simulink model "model"  (R2014a)
settings: Solver=FixedStepDiscrete  StartTime=0.0  StopTime=10  RelTol=1e-3
values from neighbouring files (symbols this model uses):
  BufLen = 4*Fs    [init_model.m]
  delay_fp1 = ceil(delay_qrs-fpdl-fpdi-fpdd)    [init_model.m]
  delay_fp2 = ceil(delay_qrs-fpdl-s)    [init_model.m]
  delay_noise = ceil(noiseds + noisedl)    [init_model.m]
  Fs = signal.fs    [init_model.m]
  s = round(0.06*Fs)    [init_model.m]
undefined symbols (not defined in the file or in its folder): fpad, fpai, fpal, fpbd, fpbi, fpbl, FrameLen, get, gopalakhermite, HR, JayMeasurePts, noiseal, noiseas, noisebl, noisebs, qrsad, qrsah, qrsai, qrsal, qrsbd, qrsbh, qrsbi, qrsbl, qrsgh, qrsgl, rochahermite1, rochahermite2, stlen
undefined symbols (not defined in the file): L1, L2, L3, L4, newL1, newL2
libraries: simulink x16, neural x14, dspbuff3 x4, dspsigops x2, dspsnks4 x1
(part 2 of 2)

== system model/Classification/Rocha Networks/Feed-Forward Neural Network/Layer 1/Delays 1 ==
  "p{1}" : Inport  PortDimensions=14  SampleTime=0.004
      mask Display: e = 0.06;c1 = [120 230 180]/255;c2 = ([120 230 180]+0)/(256+128);c3 = ([120 230 180]+128)/(256+128);patch([0 1 1 0],[0 0 1 1],c1);patch([0 1 1 1-e 1-e 0+e],[0 0 1 1-e 0+e 0+e],c2);patch([0 0 1 1-e 0+e 0+e],[0 1 1 1-e 1-e 0+e],c3);plot([0 1 1 0 0],[0 0 1 1 0]);
  mux : Mux  Inputs=1
      mask Display: e = 0.06;c1 = [120 150 230]/255;c2 = ([120 150 230]+0)/383;c3 = ([120 150 230]+128)/383;patch([0 1 1 0],[0 0 1 1],c1);patch([0 1 1 1-e 1-e 0+e],[0 0 1 1-e 0+e 0+e],c2);patch([0 0 1 1-e 0+e 0+e],[0 1 1 1-e 1-e 0+e],c3);plot([0 1 1 0 0],[0 0 1 1 0]);disp('Mux')
  "pd{1,1}" : Outport
      mask Display: e = 0.06;c1 = [120 230 180]/255;c2 = ([120 230 180]+0)/(256+128);c3 = ([120 230 180]+128)/(256+128);patch([0 1 1 0],[0 0 1 1],c1);patch([0 1 1 1-e 1-e 0+e],[0 0 1 1-e 0+e 0+e],c2);patch([0 0 1 1-e 0+e 0+e],[0 1 1 1-e 1-e 0+e],c3);plot([0 1 1 0 0],[0 0 1 1 0]);
  wires:
  mux/1 -> "pd{1,1}"/1
  "p{1}"/1 -> mux/1

== system model/Classification/Rocha Networks/Feed-Forward Neural Network/Layer 1/IW{1,1} ==
  "pd{1,1}" : Inport  PortDimensions=14  SampleTime=0.004
      mask Display: e = 0.06;c1 = [120 230 180]/255;c2 = ([120 230 180]+0)/(256+128);c3 = ([120 230 180]+128)/(256+128);patch([0 1 1 0],[0 0 1 1],c1);patch([0 1 1 1-e 1-e 0+e],[0 0 1 1-e 0+e 0+e],c2);patch([0 0 1 1-e 0+e 0+e],[0 1 1 1-e 1-e 0+e],c3);plot([0 1 1 0 0],[0 0 1 1 0]);
  "IW{1,1}(1,:)'" : Constant  Value=[-0.94852743044432697;0.20440062307916493;0.12975491445977652;-0.06056239618675234;0.069962133679617386;-0.10885123721830199;0.25849498473889437;-0.053514204484363927;-0.25705609193888052;-0.26702768869811228;-0.044345977422213696;-0.355114180368993;0.3456890098950946;0.33374461628287727]
      mask Display: e = 0.06;c1 = [120 150 230]/255;c2 = ([120 150 230]+0)/383;c3 = ([120 150 230]+128)/383;patch([0 1 1 0],[0 0 1 1],c1);patch([0 1 1 1-e 1-e 0+e],[0 0 1 1-e 0+e 0+e],c2);patch([0 0 1 1-e 0+e 0+e],[0 1 1 1-e 1-e 0+e],c3);plot([0 1 1 0 0],[0 0 1 1 0]);disp('Weights');
  "IW{1,1}(2,:)'" : Constant  Value=[4.196215953221297;-1.0964533347848004;-1.6910456916650782;1.1678044277703084;-0.91890034705408374;-1.3729579966623704;-1.6439744697625485;-1.20511805638854;-7.3755359553788633;2.9486890292671837;2.0933673220936755;-1.7229669045940939;5.0896314895005839;2.1588793540686324]
      mask Display: e = 0.06;c1 = [120 150 230]/255;c2 = ([120 150 230]+0)/383;c3 = ([120 150 230]+128)/383;patch([0 1 1 0],[0 0 1 1],c1);patch([0 1 1 1-e 1-e 0+e],[0 0 1 1-e 0+e 0+e],c2);patch([0 0 1 1-e 0+e 0+e],[0 1 1 1-e 1-e 0+e],c3);plot([0 1 1 0 0],[0 0 1 1 0]);disp('Weights');
  "IW{1,1}(3,:)'" : Constant  Value=[-119.48893768603425;100.34105004135291;-30.003324500089562;-35.099277290990273;-53.005837073603445;50.742281662417867;-89.637475943048045;20.647748261081514;-41.338537083861603;-272.57547073663108;116.09637700457249;-23.032516013581716;83.319718635034363;79.324095644747445]
      mask Display: e = 0.06;c1 = [120 150 230]/255;c2 = ([120 150 230]+0)/383;c3 = ([120 150 230]+128)/383;patch([0 1 1 0],[0 0 1 1],c1);patch([0 1 1 1-e 1-e 0+e],[0 0 1 1-e 0+e 0+e],c2);patch([0 0 1 1-e 0+e 0+e],[0 1 1 1-e 1-e 0+e],c3);plot([0 1 1 0 0],[0 0 1 1 0]);disp('Weights');
  "IW{1,1}(4,:)'" : Constant  Value=[-4.3018750079772516;-2.186870941504425;0.96285167042811259;-1.5509662850111088;0.22158991894876751;6.294576096390017;2.2813745598300921;0.037431749496884881;2.2399179091379993;4.0082296894214533;-3.678340235304538;4.351902898813651;-4.1844711515053179;-5.2925731375584135]
      mask Display: e = 0.06;c1 = [120 150 230]/255;c2 = ([120 150 230]+0)/383;c3 = ([120 150 230]+128)/383;patch([0 1 1 0],[0 0 1 1],c1);patch([0 1 1 1-e 1-e 0+e],[0 0 1 1-e 0+e 0+e],c2);patch([0 0 1 1-e 0+e 0+e],[0 1 1 1-e 1-e 0+e],c3);plot([0 1 1 0 0],[0 0 1 1 0]);disp('Weights');
  "IW{1,1}(5,:)'" : Constant  Value=[-4.8726489871410736;4.1995693373368299;1.4599627510659119;0.055179155308998161;1.0804704626757087;2.3100424258065835;2.1157870545034156;-0.12573641652203521;-8.1868510957725533;-1.5763495983381031;1.8843617318763302;-1.605559269252977;5.2697009336495135;-3.0203736798217395]
      mask Display: e = 0.06;c1 = [120 150 230]/255;c2 = ([120 150 230]+0)/383;c3 = ([120 150 230]+128)/383;patch([0 1 1 0],[0 0 1 1],c1);patch([0 1 1 1-e 1-e 0+e],[0 0 1 1-e 0+e 0+e],c2);patch([0 0 1 1-e 0+e 0+e],[0 1 1 1-e 1-e 0+e],c3);plot([0 1 1 0 0],[0 0 1 1 0]);disp('Weights');
  Mux : Mux  Inputs=5
      mask Display: e = 0.06;c1 = [120 150 230]/255;c2 = ([120 150 230]+0)/383;c3 = ([120 150 230]+128)/383;patch([0 1 1 0],[0 0 1 1],c1);patch([0 1 1 1-e 1-e 0+e],[0 0 1 1-e 0+e 0+e],c2);patch([0 0 1 1-e 0+e 0+e],[0 1 1 1-e 1-e 0+e],c3);plot([0 1 1 0 0],[0 0 1 1 0]);disp('Mux');
  dotprod{1..5} (5 alike) : neural/Weight Functions/dotprod
  "iz{1,1}" : Outport
      mask Display: e = 0.06;c1 = [120 230 180]/255;c2 = ([120 230 180]+0)/(256+128);c3 = ([120 230 180]+128)/(256+128);patch([0 1 1 0],[0 0 1 1],c1);patch([0 1 1 1-e 1-e 0+e],[0 0 1 1-e 0+e 0+e],c2);patch([0 0 1 1-e 0+e 0+e],[0 1 1 1-e 1-e 0+e],c3);plot([0 1 1 0 0],[0 0 1 1 0]);
  wires:
  Mux/1 -> "iz{1,1}"/1
  dotprod5/1 -> Mux/5
  "IW{1,1}(5,:)'"/1 -> dotprod5/1
  dotprod4/1 -> Mux/4
  "IW{1,1}(4,:)'"/1 -> dotprod4/1
  dotprod3/1 -> Mux/3
  "IW{1,1}(3,:)'"/1 -> dotprod3/1
  dotprod2/1 -> Mux/2
  "IW{1,1}(2,:)'"/1 -> dotprod2/1
  dotprod1/1 -> Mux/1
  "pd{1,1}"/1 -> dotprod5/2, dotprod4/2, dotprod3/2, dotprod2/2, dotprod1/2
  "IW{1,1}(1,:)'"/1 -> dotprod1/1

== system model/Classification/Rocha Networks/Feed-Forward Neural Network/Layer 2/Delays 1 ==
  "p{2}" : Inport  PortDimensions=5  SampleTime=0.004
      mask Display: e = 0.06;c1 = [120 230 180]/255;c2 = ([120 230 180]+0)/(256+128);c3 = ([120 230 180]+128)/(256+128);patch([0 1 1 0],[0 0 1 1],c1);patch([0 1 1 1-e 1-e 0+e],[0 0 1 1-e 0+e 0+e],c2);patch([0 0 1 1-e 0+e 0+e],[0 1 1 1-e 1-e 0+e],c3);plot([0 1 1 0 0],[0 0 1 1 0]);
  mux : Mux  Inputs=1
      mask Display: e = 0.06;c1 = [120 150 230]/255;c2 = ([120 150 230]+0)/383;c3 = ([120 150 230]+128)/383;patch([0 1 1 0],[0 0 1 1],c1);patch([0 1 1 1-e 1-e 0+e],[0 0 1 1-e 0+e 0+e],c2);patch([0 0 1 1-e 0+e 0+e],[0 1 1 1-e 1-e 0+e],c3);plot([0 1 1 0 0],[0 0 1 1 0]);disp('Mux')
  "pd{2,1}" : Outport
      mask Display: e = 0.06;c1 = [120 230 180]/255;c2 = ([120 230 180]+0)/(256+128);c3 = ([120 230 180]+128)/(256+128);patch([0 1 1 0],[0 0 1 1],c1);patch([0 1 1 1-e 1-e 0+e],[0 0 1 1-e 0+e 0+e],c2);patch([0 0 1 1-e 0+e 0+e],[0 1 1 1-e 1-e 0+e],c3);plot([0 1 1 0 0],[0 0 1 1 0]);
  wires:
  mux/1 -> "pd{2,1}"/1
  "p{2}"/1 -> mux/1

== system model/Classification/Rocha Networks/Feed-Forward Neural Network/Layer 2/LW{2,1} ==
  "ad{2,1}" : Inport  PortDimensions=5  SampleTime=0.004
      mask Display: e = 0.06;c1 = [120 230 180]/255;c2 = ([120 230 180]+0)/(256+128);c3 = ([120 230 180]+128)/(256+128);patch([0 1 1 0],[0 0 1 1],c1);patch([0 1 1 1-e 1-e 0+e],[0 0 1 1-e 0+e 0+e],c2);patch([0 0 1 1-e 0+e 0+e],[0 1 1 1-e 1-e 0+e],c3);plot([0 1 1 0 0],[0 0 1 1 0]);
  "IW{2,1}(1,:)'" : Constant  Value=[-149.09638162192093;367.91909524859904;-51.737357690785181;251.01905323949171;122.37984158883808]
      mask Display: e = 0.06;c1 = [120 150 230]/255;c2 = ([120 150 230]+0)/383;c3 = ([120 150 230]+128)/383;patch([0 1 1 0],[0 0 1 1],c1);patch([0 1 1 1-e 1-e 0+e],[0 0 1 1-e 0+e 0+e],c2);patch([0 0 1 1-e 0+e 0+e],[0 1 1 1-e 1-e 0+e],c3);plot([0 1 1 0 0],[0 0 1 1 0]);disp('weights');
  "IW{2,1}(2,:)'" : Constant  Value=[193.01482116073518;2.01637862811531;2.0295689251261515;2.6358537534872188;-3.0272550047565128]
      mask Display: e = 0.06;c1 = [120 150 230]/255;c2 = ([120 150 230]+0)/383;c3 = ([120 150 230]+128)/383;patch([0 1 1 0],[0 0 1 1],c1);patch([0 1 1 1-e 1-e 0+e],[0 0 1 1-e 0+e 0+e],c2);patch([0 0 1 1-e 0+e 0+e],[0 1 1 1-e 1-e 0+e],c3);plot([0 1 1 0 0],[0 0 1 1 0]);disp('weights');
  "IW{2,1}(3,:)'" : Constant  Value=[235.11702144206401;-3.2480719290191273;-470.03072596851348;-520.07693018468831;-79.123881642492648]
      mask Display: e = 0.06;c1 = [120 150 230]/255;c2 = ([120 150 230]+0)/383;c3 = ([120 150 230]+128)/383;patch([0 1 1 0],[0 0 1 1],c1);patch([0 1 1 1-e 1-e 0+e],[0 0 1 1-e 0+e 0+e],c2);patch([0 0 1 1-e 0+e 0+e],[0 1 1 1-e 1-e 0+e],c3);plot([0 1 1 0 0],[0 0 1 1 0]);disp('weights');
  Mux : Mux  Inputs=3
      mask Display: e = 0.06;c1 = [120 150 230]/255;c2 = ([120 150 230]+0)/383;c3 = ([120 150 230]+128)/383;patch([0 1 1 0],[0 0 1 1],c1);patch([0 1 1 1-e 1-e 0+e],[0 0 1 1-e 0+e 0+e],c2);patch([0 0 1 1-e 0+e 0+e],[0 1 1 1-e 1-e 0+e],c3);plot([0 1 1 0 0],[0 0 1 1 0]);disp('Mux');
  dotprod1 : neural/Weight Functions/dotprod
  dotprod2 : neural/Weight Functions/dotprod
  dotprod3 : neural/Weight Functions/dotprod
  "lz{2,1}" : Outport
      mask Display: e = 0.06;c1 = [120 230 180]/255;c2 = ([120 230 180]+0)/(256+128);c3 = ([120 230 180]+128)/(256+128);patch([0 1 1 0],[0 0 1 1],c1);patch([0 1 1 1-e 1-e 0+e],[0 0 1 1-e 0+e 0+e],c2);patch([0 0 1 1-e 0+e 0+e],[0 1 1 1-e 1-e 0+e],c3);plot([0 1 1 0 0],[0 0 1 1 0]);
  wires:
  Mux/1 -> "lz{2,1}"/1
  dotprod3/1 -> Mux/3
  "IW{2,1}(3,:)'"/1 -> dotprod3/1
  dotprod2/1 -> Mux/2
  "IW{2,1}(2,:)'"/1 -> dotprod2/1
  dotprod1/1 -> Mux/1
  "ad{2,1}"/1 -> dotprod3/2, dotprod2/2, dotprod1/2
  "IW{2,1}(1,:)'"/1 -> dotprod1/1

== system model/Classification/Rocha Networks/Feed-Forward Neural Network/Layer 3/Delays 1 ==
  "p{3}" : Inport  PortDimensions=3  SampleTime=0.004
      mask Display: e = 0.06;c1 = [120 230 180]/255;c2 = ([120 230 180]+0)/(256+128);c3 = ([120 230 180]+128)/(256+128);patch([0 1 1 0],[0 0 1 1],c1);patch([0 1 1 1-e 1-e 0+e],[0 0 1 1-e 0+e 0+e],c2);patch([0 0 1 1-e 0+e 0+e],[0 1 1 1-e 1-e 0+e],c3);plot([0 1 1 0 0],[0 0 1 1 0]);
  mux : Mux  Inputs=1
      mask Display: e = 0.06;c1 = [120 150 230]/255;c2 = ([120 150 230]+0)/383;c3 = ([120 150 230]+128)/383;patch([0 1 1 0],[0 0 1 1],c1);patch([0 1 1 1-e 1-e 0+e],[0 0 1 1-e 0+e 0+e],c2);patch([0 0 1 1-e 0+e 0+e],[0 1 1 1-e 1-e 0+e],c3);plot([0 1 1 0 0],[0 0 1 1 0]);disp('Mux')
  "pd{3,2}" : Outport
      mask Display: e = 0.06;c1 = [120 230 180]/255;c2 = ([120 230 180]+0)/(256+128);c3 = ([120 230 180]+128)/(256+128);patch([0 1 1 0],[0 0 1 1],c1);patch([0 1 1 1-e 1-e 0+e],[0 0 1 1-e 0+e 0+e],c2);patch([0 0 1 1-e 0+e 0+e],[0 1 1 1-e 1-e 0+e],c3);plot([0 1 1 0 0],[0 0 1 1 0]);
  wires:
  mux/1 -> "pd{3,2}"/1
  "p{3}"/1 -> mux/1

== system model/Classification/Rocha Networks/Feed-Forward Neural Network/Layer 3/LW{3,2} ==
  "ad{3,2}" : Inport  PortDimensions=3  SampleTime=0.004
      mask Display: e = 0.06;c1 = [120 230 180]/255;c2 = ([120 230 180]+0)/(256+128);c3 = ([120 230 180]+128)/(256+128);patch([0 1 1 0],[0 0 1 1],c1);patch([0 1 1 1-e 1-e 0+e],[0 0 1 1-e 0+e 0+e],c2);patch([0 0 1 1-e 0+e 0+e],[0 1 1 1-e 1-e 0+e],c3);plot([0 1 1 0 0],[0 0 1 1 0]);
  "IW{3,2}(1,:)'" : Constant  Value=[-0.048722154231108962;-0.87512218154191901;-0.044843737985613252]
      mask Display: e = 0.06;c1 = [120 150 230]/255;c2 = ([120 150 230]+0)/383;c3 = ([120 150 230]+128)/383;patch([0 1 1 0],[0 0 1 1],c1);patch([0 1 1 1-e 1-e 0+e],[0 0 1 1-e 0+e 0+e],c2);patch([0 0 1 1-e 0+e 0+e],[0 1 1 1-e 1-e 0+e],c3);plot([0 1 1 0 0],[0 0 1 1 0]);disp('weights');
  Mux : Mux  Inputs=1
      mask Display: e = 0.06;c1 = [120 150 230]/255;c2 = ([120 150 230]+0)/383;c3 = ([120 150 230]+128)/383;patch([0 1 1 0],[0 0 1 1],c1);patch([0 1 1 1-e 1-e 0+e],[0 0 1 1-e 0+e 0+e],c2);patch([0 0 1 1-e 0+e 0+e],[0 1 1 1-e 1-e 0+e],c3);plot([0 1 1 0 0],[0 0 1 1 0]);disp('Mux');
  dotprod1 : neural/Weight Functions/dotprod
  "lz{3,2}" : Outport
      mask Display: e = 0.06;c1 = [120 230 180]/255;c2 = ([120 230 180]+0)/(256+128);c3 = ([120 230 180]+128)/(256+128);patch([0 1 1 0],[0 0 1 1],c1);patch([0 1 1 1-e 1-e 0+e],[0 0 1 1-e 0+e 0+e],c2);patch([0 0 1 1-e 0+e 0+e],[0 1 1 1-e 1-e 0+e],c3);plot([0 1 1 0 0],[0 0 1 1 0]);
  wires:
  Mux/1 -> "lz{3,2}"/1
  dotprod1/1 -> Mux/1
  "ad{3,2}"/1 -> dotprod1/2
  "IW{3,2}(1,:)'"/1 -> dotprod1/1

== system model/Features Extraction/Mohebbi Features/Exttract ST difference/Extract ST segment/edge limits ==
  idx : Inport
  Constant1 : Constant  Value=searchL1  OutDataTypeStr=int32
  Constant2 : Constant  Value=searchL2  OutDataTypeStr=int32
  Sum : Sum  Inputs=++|
  Sum1 : Sum  Inputs=|++
  start : Outport
  end : Outport  Port=2
  def : Outport  Port=3
  wires:
  Sum1/1 -> start/1
  Sum/1 -> end/1
  Constant2/1 -> Sum/2
  Constant1/1 -> Sum1/1
  idx/1 -> Sum1/2, Sum/1, def/1

== system model/Preprocessing/Subsystem/FP Detection/Detect P wave points/Search onset and offset ==
  buffM : Inport
  peak : Inport  Port=2
  Check Polarity : Subsystem  mask{BufferLength=BufLen}
      mask prompts: BufferLength "Buffer length"
  Inverted wave : Subsystem
  Logical Operator : Logic  Operator=NOT  AllPortsSameDT=off  OutDataTypeStr=boolean
  Normal wave : Subsystem
  Switch : Switch  Criteria=u2 > Threshold
  Switch1 : Switch  Criteria=u2 > Threshold
  onset : Outport
  offset : Outport  Port=2
  wires:
  peak/1 -> Inverted wave/2(peak), Check Polarity/2(idx), Normal wave/2(peak)
  buffM/1 -> Normal wave/1(buffM), Check Polarity/1(buf), Inverted wave/1(buffM)
  Check Polarity/1(inv) -> Inverted wave/Enable, Logical Operator/1
  Logical Operator/1 -> Switch1/2, Normal wave/Enable, Switch/2
  Normal wave/1(onset) -> Switch/1
  Switch/1 -> onset/1
  Switch1/1 -> offset/1
  Inverted wave/2(offset) -> Switch1/3
  Inverted wave/1(onset) -> Switch/3
  Normal wave/2(offset) -> Switch1/1

== system model/Preprocessing/Subsystem/FP Detection/Detect P wave points/peak limits ==
  idx : Inport
  len : Inport  Port=2
  Constant1 : Constant  Value=searchL1  OutDataTypeStr=int32
  Gain : Gain  Gain=searchL2Mult  OutDataTypeStr=int32
  Sum : Sum  Inputs=++|
  Sum1 : Sum  Inputs=|++
  start : Outport
  end : Outport  Port=2
  def : Outport  Port=3
  wires:
  Sum1/1 -> start/1
  Sum/1 -> end/1
  Constant1/1 -> Sum1/1
  idx/1 -> Sum1/2, Sum/1, def/1
  Gain/1 -> Sum/2
  len/1 -> Gain/1

== system model/Preprocessing/Subsystem/FP Detection/Detect R wave points/Search onset and offset ==
  buffM : Inport
  peak : Inport  Port=2
  Check Polarity : Subsystem  mask{BufferLength=BufLen}
      mask prompts: BufferLength "Buffer length"
  Inverted wave : Subsystem
  Logical Operator : Logic  Operator=NOT  AllPortsSameDT=off  OutDataTypeStr=boolean
  Normal wave : Subsystem
  Switch : Switch  Criteria=u2 > Threshold
  Switch1 : Switch  Criteria=u2 > Threshold
  onset : Outport
  offset : Outport  Port=2
  wires:
  Switch1/1 -> offset/1
  Switch/1 -> onset/1
  Logical Operator/1 -> Switch1/2, Normal wave/Enable, Switch/2
  Normal wave/2(offset) -> Switch1/1
  Check Polarity/1(inv) -> Inverted wave/Enable, Logical Operator/1
  buffM/1 -> Inverted wave/1(buffM), Check Polarity/1(buf), Normal wave/1(buffM)
  peak/1 -> Inverted wave/2(peak), Normal wave/2(peak), Check Polarity/2(idx)
  Normal wave/1(onset) -> Switch/1
  Inverted wave/2(offset) -> Switch1/3
  Inverted wave/1(onset) -> Switch/3

== system model/Preprocessing/Subsystem/FP Detection/Detect R wave points/peak limits ==
  idx : Inport
  Constant1 : Constant  Value=searchL1  OutDataTypeStr=int32
  Constant2 : Constant  Value=searchL2  OutDataTypeStr=int32
  Sum : Sum  Inputs=++|
  Sum1 : Sum  Inputs=|++
  start : Outport
  end : Outport  Port=2
  def : Outport  Port=3
  wires:
  idx/1 -> def/1, Sum/1, Sum1/2
  Constant1/1 -> Sum1/1
  Constant2/1 -> Sum/2
  Sum/1 -> end/1
  Sum1/1 -> start/1

== system model/Preprocessing/Subsystem/FP Detection/Detect T wave points/Search onset and offset ==
  buffM : Inport
  peak : Inport  Port=2
  Check Polarity : Subsystem  mask{BufferLength=BufLen}
      mask prompts: BufferLength "Buffer length"
  Inverted wave : Subsystem
  Logical Operator : Logic  Operator=NOT  AllPortsSameDT=off  OutDataTypeStr=boolean
  Normal wave : Subsystem
  Switch : Switch  Criteria=u2 > Threshold
  Switch1 : Switch  Criteria=u2 > Threshold
  onset : Outport
  offset : Outport  Port=2
  wires:
  Normal wave/2(offset) -> Switch1/1
  Inverted wave/1(onset) -> Switch/3
  Inverted wave/2(offset) -> Switch1/3
  Switch1/1 -> offset/1
  Switch/1 -> onset/1
  Normal wave/1(onset) -> Switch/1
  Logical Operator/1 -> Switch/2, Normal wave/Enable, Switch1/2
  Check Polarity/1(inv) -> Logical Operator/1, Inverted wave/Enable
  buffM/1 -> Check Polarity/1(buf), Inverted wave/1(buffM), Normal wave/1(buffM)
  peak/1 -> Check Polarity/2(idx), Normal wave/2(peak), Inverted wave/2(peak)

== system model/Preprocessing/Subsystem/FP Detection/Detect T wave points/peak limits ==
  idx : Inport
  len : Inport  Port=2
  Constant1 : Constant  Value=searchL1  OutDataTypeStr=int32
  Gain : Gain  Gain=searchL2Mult  OutDataTypeStr=int32
  Sum : Sum  Inputs=++|
  Sum1 : Sum  Inputs=|++
  start : Outport
  end : Outport  Port=2
  def : Outport  Port=3
  wires:
  len/1 -> Gain/1
  Gain/1 -> Sum/2
  idx/1 -> def/1, Sum/1, Sum1/2
  Constant1/1 -> Sum1/1
  Sum/1 -> end/1
  Sum1/1 -> start/1

== system model/Preprocessing/Subsystem/QRS Detection/Evaluate Peaks/Peak Selector ==
  CurrIdx : Inport
  SbackIdx : Inport  Port=2
  Compare To Zero : simulink/Logic and Bit Operations/Compare To Zero  relop=~=  OutDataTypeStr=boolean
  Switch1 : Switch  Criteria=u2 ~= 0  OutDataTypeStr=int32
  PeakIdx : Outport
  Searchback : Outport  Port=2
  wires:
  Switch1/1 -> PeakIdx/1
  CurrIdx/1 -> Switch1/3
  SbackIdx/1 -> Compare To Zero/1, Switch1/2, Switch1/1
  Compare To Zero/1 -> Searchback/1

== system model/Preprocessing/Subsystem/QRS Detection/Evaluate Peaks/Threshold ==
  Signal : Inport
  Noise : Inport  Port=2
  Abs : Abs  OutDataTypeStr=int32
  Constant2 : Constant  Value=4  OutDataTypeStr=int32
  Divide : Product  Inputs=*/  OutDataTypeStr=int32
  Sum : Sum  Inputs=|++  AccumDataTypeStr=int32  OutDataTypeStr=int32
  Sum1 : Sum  Inputs=|++  AccumDataTypeStr=int32  OutDataTypeStr=int32
  Thresh : Outport
  wires:
  Constant2/1 -> Divide/2
  Signal/1 -> Sum/1
  Noise/1 -> Sum/2, Sum1/2
  Sum/1 -> Abs/1
  Abs/1 -> Divide/1
  Sum1/1 -> Thresh/1
  Divide/1 -> Sum1/1

== system model/Preprocessing/Subsystem/QRS Detection/Evaluate Peaks/Validate ==
  Detected : Inport
  Training : Inport  Port=2
  Logical Operator : Logic  AllPortsSameDT=off  OutDataTypeStr=boolean
  Logical Operator1 : Logic  Operator=NOT  AllPortsSameDT=off  OutDataTypeStr=boolean
  Valid : Outport
  wires:
  Logical Operator1/1 -> Logical Operator/2
  Detected/1 -> Logical Operator/1
  Logical Operator/1 -> Valid/1
  Training/1 -> Logical Operator1/1

== system model/Preprocessing/Subsystem/FP Detection/Detect P wave points/Search onset and offset/Check Polarity ==
  buf : Inport
  idx : Inport  Port=2
  Compare To Zero : simulink/Logic and Bit Operations/Compare To Zero  relop=>  OutDataTypeStr=boolean
  Constant : Constant  Value=BufferLength
  Selector : Selector  InputPortWidth=BufferLength  IndexOptions=Index vector (port)  Indices=[1 3]
  Sum : Sum  Inputs=|++
  inv : Outport
  wires:
  idx/1 -> Sum/1
  buf/1 -> Selector/1
  Constant/1 -> Sum/2
  Compare To Zero/1 -> inv/1
  Sum/1 -> Selector/2
  Selector/1 -> Compare To Zero/1

== system model/Preprocessing/Subsystem/FP Detection/Detect P wave points/Search onset and offset/Inverted wave ==
  buffM : Inport
  peak : Inport  Port=2
  Enable : EnablePort
  Search offset : S-Function  FunctionName=msfcn_searchbest  Parameters=Fs false  EnableBusSupport=off
  Search onset : S-Function  FunctionName=msfcn_searchbest  Parameters=Fs false  EnableBusSupport=off
  offset limits : Subsystem  mask{searchL1=1, searchL2=L3}
      mask prompts: searchL1 "First search offset (in samples)"; searchL2 "Second search offset (in samples)"
  onset limits : Subsystem  mask{searchL1=-1, searchL2=-L3}
      mask prompts: searchL1 "First search offset (in samples)"; searchL2 "Second search offset (in samples)"
  onset : Outport
  offset : Outport  Port=2
  wires:
  Search onset/1 -> onset/1
  Search offset/1 -> offset/1
  buffM/1 -> Search onset/1, Search offset/1
  onset limits/1(start) -> Search onset/2
  onset limits/2(end) -> Search onset/3
  onset limits/3(def) -> Search onset/4
  offset limits/3(def) -> Search offset/4
  offset limits/2(end) -> Search offset/3
  offset limits/1(start) -> Search offset/2
  peak/1 -> offset limits/1(idx), onset limits/1(idx)

== system model/Preprocessing/Subsystem/FP Detection/Detect P wave points/Search onset and offset/Normal wave ==
  buffM : Inport
  peak : Inport  Port=2
  Enable : EnablePort
  Search offset : S-Function  FunctionName=msfcn_searchbest  Parameters=Fs true  EnableBusSupport=off
  Search onset : S-Function  FunctionName=msfcn_searchbest  Parameters=Fs true  EnableBusSupport=off
  offset limits : Subsystem  mask{searchL1=1, searchL2=L3}
      mask prompts: searchL1 "First search offset (in samples)"; searchL2 "Second search offset (in samples)"
  onset limits : Subsystem  mask{searchL1=-1, searchL2=-L3}
      mask prompts: searchL1 "First search offset (in samples)"; searchL2 "Second search offset (in samples)"
  onset : Outport
  offset : Outport  Port=2
  wires:
  peak/1 -> onset limits/1(idx), offset limits/1(idx)
  offset limits/1(start) -> Search offset/2
  offset limits/2(end) -> Search offset/3
  offset limits/3(def) -> Search offset/4
  onset limits/3(def) -> Search onset/4
  onset limits/2(end) -> Search onset/3
  onset limits/1(start) -> Search onset/2
  buffM/1 -> Search offset/1, Search onset/1
  Search offset/1 -> offset/1
  Search onset/1 -> onset/1

== system model/Preprocessing/Subsystem/FP Detection/Detect R wave points/Search onset and offset/Check Polarity ==
  buf : Inport
  idx : Inport  Port=2
  Compare To Zero : simulink/Logic and Bit Operations/Compare To Zero  relop=>  OutDataTypeStr=boolean
  Constant : Constant  Value=BufferLength
  Selector : Selector  InputPortWidth=BufferLength  IndexOptions=Index vector (port)  Indices=[1 3]
  Sum : Sum  Inputs=|++
  inv : Outport
  wires:
  idx/1 -> Sum/1
  buf/1 -> Selector/1
  Constant/1 -> Sum/2
  Compare To Zero/1 -> inv/1
  Sum/1 -> Selector/2
  Selector/1 -> Compare To Zero/1

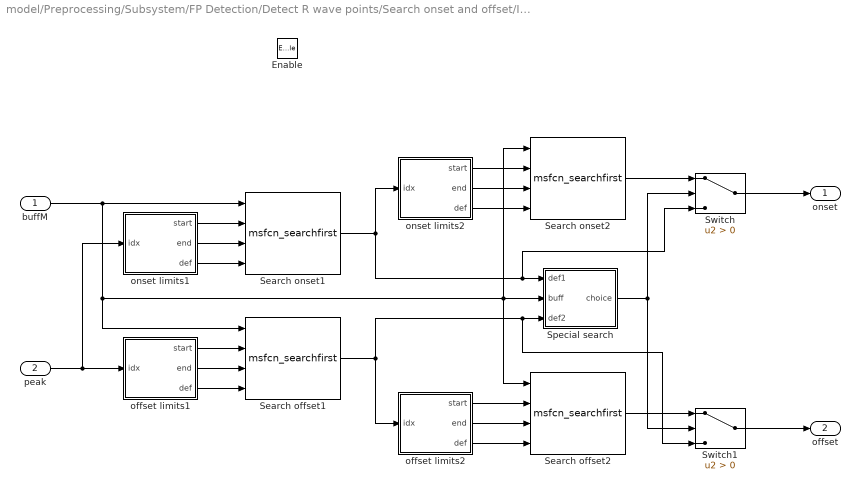
== system model/Preprocessing/Subsystem/FP Detection/Detect R wave points/Search onset and offset/Inverted wave ==
  buffM : Inport
  peak : Inport  Port=2
  Enable : EnablePort
  Search offset1 : S-Function  FunctionName=msfcn_searchfirst  Parameters=Fs true  EnableBusSupport=off
  Search offset2 : S-Function  FunctionName=msfcn_searchfirst  Parameters=Fs false  EnableBusSupport=off
  Search onset1 : S-Function  FunctionName=msfcn_searchfirst  Parameters=Fs true  EnableBusSupport=off
  Search onset2 : S-Function  FunctionName=msfcn_searchfirst  Parameters=Fs false  EnableBusSupport=off
  Special search : Subsystem
  Switch : Switch  Criteria=u2 > Threshold
  Switch1 : Switch  Criteria=u2 > Threshold
  offset limits1 : Subsystem  mask{searchL1=L2, searchL2=L1}
      mask prompts: searchL1 "First search offset (in samples)"; searchL2 "Second search offset (in samples)"
  offset limits2 : Subsystem  mask{searchL1=1, searchL2=L4}
      mask prompts: searchL1 "First search offset (in samples)"; searchL2 "Second search offset (in samples)"
  onset limits1 : Subsystem  mask{searchL1=-L2, searchL2=-L1}
      mask prompts: searchL1 "First search offset (in samples)"; searchL2 "Second search offset (in samples)"
  onset limits2 : Subsystem  mask{searchL1=-1, searchL2=-L4}
      mask prompts: searchL1 "First search offset (in samples)"; searchL2 "Second search offset (in samples)"
  onset : Outport
  offset : Outport  Port=2
  wires:
  Search offset2/1 -> Switch1/1
  Special search/1(choice) -> Switch/2, Switch1/2
  Search onset2/1 -> Switch/1
  Search offset1/1 -> Special search/3(def2), Switch1/3, offset limits2/1(idx)
  Search onset1/1 -> Special search/1(def1), Switch/3, onset limits2/1(idx)
  Switch1/1 -> offset/1
  Switch/1 -> onset/1
  peak/1 -> offset limits1/1(idx), onset limits1/1(idx)
  offset limits1/1(start) -> Search offset1/2
  offset limits1/2(end) -> Search offset1/3
  offset limits1/3(def) -> Search offset1/4
  onset limits1/3(def) -> Search onset1/4
  onset limits1/2(end) -> Search onset1/3
  onset limits1/1(start) -> Search onset1/2
  offset limits2/3(def) -> Search offset2/4
  offset limits2/2(end) -> Search offset2/3
  offset limits2/1(start) -> Search offset2/2
  onset limits2/3(def) -> Search onset2/4
  onset limits2/2(end) -> Search onset2/3
  onset limits2/1(start) -> Search onset2/2
  buffM/1 -> Search onset1/1, Search onset2/1, Search offset2/1, Special search/2(buff), Search offset1/1

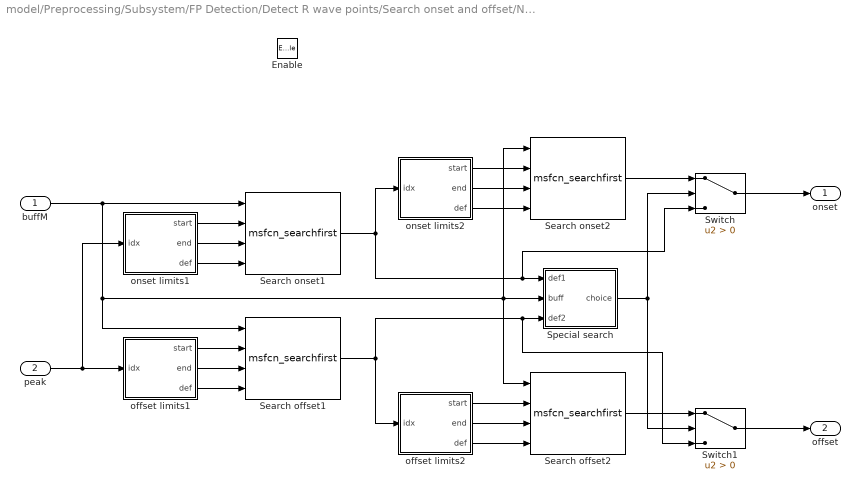
== system model/Preprocessing/Subsystem/FP Detection/Detect R wave points/Search onset and offset/Normal wave ==
  buffM : Inport
  peak : Inport  Port=2
  Enable : EnablePort
  Search offset1 : S-Function  FunctionName=msfcn_searchfirst  Parameters=Fs true  EnableBusSupport=off
  Search offset2 : S-Function  FunctionName=msfcn_searchfirst  Parameters=Fs false  EnableBusSupport=off
  Search onset1 : S-Function  FunctionName=msfcn_searchfirst  Parameters=Fs true  EnableBusSupport=off
  Search onset2 : S-Function  FunctionName=msfcn_searchfirst  Parameters=Fs false  EnableBusSupport=off
  Special search : Subsystem
  Switch : Switch  Criteria=u2 > Threshold
  Switch1 : Switch  Criteria=u2 > Threshold
  offset limits1 : Subsystem  mask{searchL1=L2, searchL2=L1}
      mask prompts: searchL1 "First search offset (in samples)"; searchL2 "Second search offset (in samples)"
  offset limits2 : Subsystem  mask{searchL1=1, searchL2=L4}
      mask prompts: searchL1 "First search offset (in samples)"; searchL2 "Second search offset (in samples)"
  onset limits1 : Subsystem  mask{searchL1=-L2, searchL2=-L1}
      mask prompts: searchL1 "First search offset (in samples)"; searchL2 "Second search offset (in samples)"
  onset limits2 : Subsystem  mask{searchL1=-1, searchL2=-L4}
      mask prompts: searchL1 "First search offset (in samples)"; searchL2 "Second search offset (in samples)"
  onset : Outport
  offset : Outport  Port=2
  wires:
  buffM/1 -> Search offset1/1, Special search/2(buff), Search offset2/1, Search onset2/1, Search onset1/1
  onset limits2/1(start) -> Search onset2/2
  onset limits2/2(end) -> Search onset2/3
  onset limits2/3(def) -> Search onset2/4
  offset limits2/1(start) -> Search offset2/2
  offset limits2/2(end) -> Search offset2/3
  offset limits2/3(def) -> Search offset2/4
  onset limits1/1(start) -> Search onset1/2
  onset limits1/2(end) -> Search onset1/3
  onset limits1/3(def) -> Search onset1/4
  offset limits1/3(def) -> Search offset1/4
  offset limits1/2(end) -> Search offset1/3
  offset limits1/1(start) -> Search offset1/2
  peak/1 -> onset limits1/1(idx), offset limits1/1(idx)
  Switch/1 -> onset/1
  Switch1/1 -> offset/1
  Search onset1/1 -> onset limits2/1(idx), Switch/3, Special search/1(def1)
  Search offset1/1 -> offset limits2/1(idx), Switch1/3, Special search/3(def2)
  Search onset2/1 -> Switch/1
  Special search/1(choice) -> Switch1/2, Switch/2
  Search offset2/1 -> Switch1/1

== system model/Preprocessing/Subsystem/FP Detection/Detect T wave points/Search onset and offset/Check Polarity ==
  buf : Inport
  idx : Inport  Port=2
  Compare To Zero : simulink/Logic and Bit Operations/Compare To Zero  relop=>  OutDataTypeStr=boolean
  Constant : Constant  Value=BufferLength
  Selector : Selector  InputPortWidth=BufferLength  IndexOptions=Index vector (port)  Indices=[1 3]
  Sum : Sum  Inputs=|++
  inv : Outport
  wires:
  idx/1 -> Sum/1
  buf/1 -> Selector/1
  Constant/1 -> Sum/2
  Compare To Zero/1 -> inv/1
  Sum/1 -> Selector/2
  Selector/1 -> Compare To Zero/1

== system model/Preprocessing/Subsystem/FP Detection/Detect T wave points/Search onset and offset/Inverted wave ==
  buffM : Inport
  peak : Inport  Port=2
  Enable : EnablePort
  Search offset : S-Function  FunctionName=msfcn_searchbest  Parameters=Fs false  EnableBusSupport=off
  Search onset : S-Function  FunctionName=msfcn_searchbest  Parameters=Fs false  EnableBusSupport=off
  offset limits : Subsystem  mask{searchL1=1, searchL2=L3}
      mask prompts: searchL1 "First search offset (in samples)"; searchL2 "Second search offset (in samples)"
  onset limits : Subsystem  mask{searchL1=-1, searchL2=-L3}
      mask prompts: searchL1 "First search offset (in samples)"; searchL2 "Second search offset (in samples)"
  onset : Outport
  offset : Outport  Port=2
  wires:
  peak/1 -> onset limits/1(idx), offset limits/1(idx)
  offset limits/1(start) -> Search offset/2
  offset limits/2(end) -> Search offset/3
  offset limits/3(def) -> Search offset/4
  onset limits/3(def) -> Search onset/4
  onset limits/2(end) -> Search onset/3
  onset limits/1(start) -> Search onset/2
  buffM/1 -> Search offset/1, Search onset/1
  Search offset/1 -> offset/1
  Search onset/1 -> onset/1

== system model/Preprocessing/Subsystem/FP Detection/Detect T wave points/Search onset and offset/Normal wave ==
  buffM : Inport
  peak : Inport  Port=2
  Enable : EnablePort
  Search offset : S-Function  FunctionName=msfcn_searchbest  Parameters=Fs true  EnableBusSupport=off
  Search onset : S-Function  FunctionName=msfcn_searchbest  Parameters=Fs true  EnableBusSupport=off
  offset limits : Subsystem  mask{searchL1=1, searchL2=L3}
      mask prompts: searchL1 "First search offset (in samples)"; searchL2 "Second search offset (in samples)"
  onset limits : Subsystem  mask{searchL1=-1, searchL2=-L3}
      mask prompts: searchL1 "First search offset (in samples)"; searchL2 "Second search offset (in samples)"
  onset : Outport
  offset : Outport  Port=2
  wires:
  Search onset/1 -> onset/1
  Search offset/1 -> offset/1
  buffM/1 -> Search onset/1, Search offset/1
  onset limits/1(start) -> Search onset/2
  onset limits/2(end) -> Search onset/3
  onset limits/3(def) -> Search onset/4
  offset limits/3(def) -> Search offset/4
  offset limits/2(end) -> Search offset/3
  offset limits/1(start) -> Search offset/2
  peak/1 -> offset limits/1(idx), onset limits/1(idx)

== system model/Preprocessing/Subsystem/FP Detection/Detect P wave points/Search onset and offset/Inverted wave/offset limits ==
  idx : Inport
  Constant1 : Constant  Value=searchL1  OutDataTypeStr=int32
  Constant2 : Constant  Value=searchL2  OutDataTypeStr=int32
  Sum : Sum  Inputs=++|
  Sum1 : Sum  Inputs=|++
  start : Outport
  end : Outport  Port=2
  def : Outport  Port=3
  wires:
  Sum1/1 -> start/1
  Sum/1 -> end/1
  Constant2/1 -> Sum/2
  Constant1/1 -> Sum1/1
  idx/1 -> Sum1/2, Sum/1, def/1

== system model/Preprocessing/Subsystem/FP Detection/Detect P wave points/Search onset and offset/Inverted wave/onset limits ==
  idx : Inport
  Constant1 : Constant  Value=searchL1  OutDataTypeStr=int32
  Constant2 : Constant  Value=searchL2  OutDataTypeStr=int32
  Sum : Sum  Inputs=++|
  Sum1 : Sum  Inputs=|++
  start : Outport
  end : Outport  Port=2
  def : Outport  Port=3
  wires:
  idx/1 -> def/1, Sum/1, Sum1/2
  Constant1/1 -> Sum1/1
  Constant2/1 -> Sum/2
  Sum/1 -> end/1
  Sum1/1 -> start/1

== system model/Preprocessing/Subsystem/FP Detection/Detect P wave points/Search onset and offset/Normal wave/offset limits ==
  idx : Inport
  Constant1 : Constant  Value=searchL1  OutDataTypeStr=int32
  Constant2 : Constant  Value=searchL2  OutDataTypeStr=int32
  Sum : Sum  Inputs=++|
  Sum1 : Sum  Inputs=|++
  start : Outport
  end : Outport  Port=2
  def : Outport  Port=3
  wires:
  idx/1 -> def/1, Sum/1, Sum1/2
  Constant1/1 -> Sum1/1
  Constant2/1 -> Sum/2
  Sum/1 -> end/1
  Sum1/1 -> start/1

== system model/Preprocessing/Subsystem/FP Detection/Detect P wave points/Search onset and offset/Normal wave/onset limits ==
  idx : Inport
  Constant1 : Constant  Value=searchL1  OutDataTypeStr=int32
  Constant2 : Constant  Value=searchL2  OutDataTypeStr=int32
  Sum : Sum  Inputs=++|
  Sum1 : Sum  Inputs=|++
  start : Outport
  end : Outport  Port=2
  def : Outport  Port=3
  wires:
  Sum1/1 -> start/1
  Sum/1 -> end/1
  Constant2/1 -> Sum/2
  Constant1/1 -> Sum1/1
  idx/1 -> Sum1/2, Sum/1, def/1

== system model/Preprocessing/Subsystem/FP Detection/Detect R wave points/Search onset and offset/Inverted wave/Special search ==
  def1 : Inport
  buff : Inport  Port=2
  def2 : Inport  Port=3
  Check Value : Subsystem  mask{BufferLength=BufLen}
      mask prompts: BufferLength "Buffer length"
  Check Value1 : Subsystem  mask{BufferLength=BufLen}
      mask prompts: BufferLength "Buffer length"
  Logical Operator : Logic  AllPortsSameDT=off  OutDataTypeStr=boolean
  Relational Operator : RelationalOperator  Operator=~=  OutDataTypeStr=boolean
  Relational Operator1 : RelationalOperator  OutDataTypeStr=boolean
  choice : Outport
  wires:
  Logical Operator/1 -> choice/1
  Check Value/1(val) -> Relational Operator1/1
  Relational Operator1/1 -> Logical Operator/1
  Check Value1/1(val) -> Relational Operator1/2
  def2/1 -> Check Value1/2(idx)
  buff/1 -> Check Value1/1(buf), Check Value/1(buf)
  def1/1 -> Check Value/2(idx)
  Relational Operator/1 -> Logical Operator/2
  Check Value/2(sign) -> Relational Operator/1
  Check Value1/2(sign) -> Relational Operator/2

== system model/Preprocessing/Subsystem/FP Detection/Detect R wave points/Search onset and offset/Inverted wave/offset limits1 ==
  idx : Inport
  Constant1 : Constant  Value=searchL1  OutDataTypeStr=int32
  Constant2 : Constant  Value=searchL2  OutDataTypeStr=int32
  Sum : Sum  Inputs=++|
  Sum1 : Sum  Inputs=|++
  start : Outport
  end : Outport  Port=2
  def : Outport  Port=3
  wires:
  idx/1 -> def/1, Sum/1, Sum1/2
  Constant1/1 -> Sum1/1
  Constant2/1 -> Sum/2
  Sum/1 -> end/1
  Sum1/1 -> start/1

== system model/Preprocessing/Subsystem/FP Detection/Detect R wave points/Search onset and offset/Inverted wave/offset limits2 ==
  idx : Inport
  Constant1 : Constant  Value=searchL1  OutDataTypeStr=int32
  Constant2 : Constant  Value=searchL2  OutDataTypeStr=int32
  Sum : Sum  Inputs=++|
  Sum1 : Sum  Inputs=|++
  start : Outport
  end : Outport  Port=2
  def : Outport  Port=3
  wires:
  Sum1/1 -> start/1
  Sum/1 -> end/1
  Constant2/1 -> Sum/2
  Constant1/1 -> Sum1/1
  idx/1 -> Sum1/2, Sum/1, def/1

== system model/Preprocessing/Subsystem/FP Detection/Detect R wave points/Search onset and offset/Inverted wave/onset limits1 ==
  idx : Inport
  Constant1 : Constant  Value=searchL1  OutDataTypeStr=int32
  Constant2 : Constant  Value=searchL2  OutDataTypeStr=int32
  Sum : Sum  Inputs=++|
  Sum1 : Sum  Inputs=|++
  start : Outport
  end : Outport  Port=2
  def : Outport  Port=3
  wires:
  Sum1/1 -> start/1
  Sum/1 -> end/1
  Constant2/1 -> Sum/2
  Constant1/1 -> Sum1/1
  idx/1 -> Sum1/2, Sum/1, def/1

== system model/Preprocessing/Subsystem/FP Detection/Detect R wave points/Search onset and offset/Inverted wave/onset limits2 ==
  idx : Inport
  Constant1 : Constant  Value=searchL1  OutDataTypeStr=int32
  Constant2 : Constant  Value=searchL2  OutDataTypeStr=int32
  Sum : Sum  Inputs=++|
  Sum1 : Sum  Inputs=|++
  start : Outport
  end : Outport  Port=2
  def : Outport  Port=3
  wires:
  idx/1 -> def/1, Sum/1, Sum1/2
  Constant1/1 -> Sum1/1
  Constant2/1 -> Sum/2
  Sum/1 -> end/1
  Sum1/1 -> start/1

== system model/Preprocessing/Subsystem/FP Detection/Detect R wave points/Search onset and offset/Normal wave/Special search ==
  def1 : Inport
  buff : Inport  Port=2
  def2 : Inport  Port=3
  Check Value : Subsystem  mask{BufferLength=BufLen}
      mask prompts: BufferLength "Buffer length"
  Check Value1 : Subsystem  mask{BufferLength=BufLen}
      mask prompts: BufferLength "Buffer length"
  Logical Operator : Logic  AllPortsSameDT=off  OutDataTypeStr=boolean
  Relational Operator : RelationalOperator  Operator=~=  OutDataTypeStr=boolean
  Relational Operator1 : RelationalOperator  OutDataTypeStr=boolean
  choice : Outport
  wires:
  Check Value1/2(sign) -> Relational Operator/2
  Check Value/2(sign) -> Relational Operator/1
  Relational Operator/1 -> Logical Operator/2
  def1/1 -> Check Value/2(idx)
  buff/1 -> Check Value1/1(buf), Check Value/1(buf)
  def2/1 -> Check Value1/2(idx)
  Check Value1/1(val) -> Relational Operator1/2
  Relational Operator1/1 -> Logical Operator/1
  Check Value/1(val) -> Relational Operator1/1
  Logical Operator/1 -> choice/1

== system model/Preprocessing/Subsystem/FP Detection/Detect R wave points/Search onset and offset/Normal wave/offset limits1 ==
  idx : Inport
  Constant1 : Constant  Value=searchL1  OutDataTypeStr=int32
  Constant2 : Constant  Value=searchL2  OutDataTypeStr=int32
  Sum : Sum  Inputs=++|
  Sum1 : Sum  Inputs=|++
  start : Outport
  end : Outport  Port=2
  def : Outport  Port=3
  wires:
  Sum1/1 -> start/1
  Sum/1 -> end/1
  Constant2/1 -> Sum/2
  Constant1/1 -> Sum1/1
  idx/1 -> Sum1/2, Sum/1, def/1

== system model/Preprocessing/Subsystem/FP Detection/Detect R wave points/Search onset and offset/Normal wave/offset limits2 ==
  idx : Inport
  Constant1 : Constant  Value=searchL1  OutDataTypeStr=int32
  Constant2 : Constant  Value=searchL2  OutDataTypeStr=int32
  Sum : Sum  Inputs=++|
  Sum1 : Sum  Inputs=|++
  start : Outport
  end : Outport  Port=2
  def : Outport  Port=3
  wires:
  idx/1 -> def/1, Sum/1, Sum1/2
  Constant1/1 -> Sum1/1
  Constant2/1 -> Sum/2
  Sum/1 -> end/1
  Sum1/1 -> start/1

== system model/Preprocessing/Subsystem/FP Detection/Detect R wave points/Search onset and offset/Normal wave/onset limits1 ==
  idx : Inport
  Constant1 : Constant  Value=searchL1  OutDataTypeStr=int32
  Constant2 : Constant  Value=searchL2  OutDataTypeStr=int32
  Sum : Sum  Inputs=++|
  Sum1 : Sum  Inputs=|++
  start : Outport
  end : Outport  Port=2
  def : Outport  Port=3
  wires:
  idx/1 -> def/1, Sum/1, Sum1/2
  Constant1/1 -> Sum1/1
  Constant2/1 -> Sum/2
  Sum/1 -> end/1
  Sum1/1 -> start/1

== system model/Preprocessing/Subsystem/FP Detection/Detect R wave points/Search onset and offset/Normal wave/onset limits2 ==
  idx : Inport
  Constant1 : Constant  Value=searchL1  OutDataTypeStr=int32
  Constant2 : Constant  Value=searchL2  OutDataTypeStr=int32
  Sum : Sum  Inputs=++|
  Sum1 : Sum  Inputs=|++
  start : Outport
  end : Outport  Port=2
  def : Outport  Port=3
  wires:
  Sum1/1 -> start/1
  Sum/1 -> end/1
  Constant2/1 -> Sum/2
  Constant1/1 -> Sum1/1
  idx/1 -> Sum1/2, Sum/1, def/1

== system model/Preprocessing/Subsystem/FP Detection/Detect T wave points/Search onset and offset/Inverted wave/offset limits ==
  idx : Inport
  Constant1 : Constant  Value=searchL1  OutDataTypeStr=int32
  Constant2 : Constant  Value=searchL2  OutDataTypeStr=int32
  Sum : Sum  Inputs=++|
  Sum1 : Sum  Inputs=|++
  start : Outport
  end : Outport  Port=2
  def : Outport  Port=3
  wires:
  idx/1 -> def/1, Sum/1, Sum1/2
  Constant1/1 -> Sum1/1
  Constant2/1 -> Sum/2
  Sum/1 -> end/1
  Sum1/1 -> start/1

== system model/Preprocessing/Subsystem/FP Detection/Detect T wave points/Search onset and offset/Inverted wave/onset limits ==
  idx : Inport
  Constant1 : Constant  Value=searchL1  OutDataTypeStr=int32
  Constant2 : Constant  Value=searchL2  OutDataTypeStr=int32
  Sum : Sum  Inputs=++|
  Sum1 : Sum  Inputs=|++
  start : Outport
  end : Outport  Port=2
  def : Outport  Port=3
  wires:
  Sum1/1 -> start/1
  Sum/1 -> end/1
  Constant2/1 -> Sum/2
  Constant1/1 -> Sum1/1
  idx/1 -> Sum1/2, Sum/1, def/1

== system model/Preprocessing/Subsystem/FP Detection/Detect T wave points/Search onset and offset/Normal wave/offset limits ==
  idx : Inport
  Constant1 : Constant  Value=searchL1  OutDataTypeStr=int32
  Constant2 : Constant  Value=searchL2  OutDataTypeStr=int32
  Sum : Sum  Inputs=++|
  Sum1 : Sum  Inputs=|++
  start : Outport
  end : Outport  Port=2
  def : Outport  Port=3
  wires:
  Sum1/1 -> start/1
  Sum/1 -> end/1
  Constant2/1 -> Sum/2
  Constant1/1 -> Sum1/1
  idx/1 -> Sum1/2, Sum/1, def/1

== system model/Preprocessing/Subsystem/FP Detection/Detect T wave points/Search onset and offset/Normal wave/onset limits ==
  idx : Inport
  Constant1 : Constant  Value=searchL1  OutDataTypeStr=int32
  Constant2 : Constant  Value=searchL2  OutDataTypeStr=int32
  Sum : Sum  Inputs=++|
  Sum1 : Sum  Inputs=|++
  start : Outport
  end : Outport  Port=2
  def : Outport  Port=3
  wires:
  idx/1 -> def/1, Sum/1, Sum1/2
  Constant1/1 -> Sum1/1
  Constant2/1 -> Sum/2
  Sum/1 -> end/1
  Sum1/1 -> start/1

== system model/Preprocessing/Subsystem/FP Detection/Detect R wave points/Search onset and offset/Inverted wave/Special search/Check Value ==
  buf : Inport
  idx : Inport  Port=2
  Abs : Abs
  Compare To Zero : simulink/Logic and Bit Operations/Compare To Zero  relop=<  OutDataTypeStr=boolean
  Constant : Constant  Value=BufferLength
  Selector : Selector  InputPortWidth=BufferLength  IndexOptions=Index vector (port)  Indices=[1 3]
  Sum : Sum  Inputs=|++
  val : Outport
  sign : Outport  Port=2
  wires:
  Sum/1 -> Selector/2
  Compare To Zero/1 -> sign/1
  Constant/1 -> Sum/2
  buf/1 -> Selector/1
  idx/1 -> Sum/1
  Abs/1 -> val/1
  Selector/1 -> Abs/1, Compare To Zero/1

== system model/Preprocessing/Subsystem/FP Detection/Detect R wave points/Search onset and offset/Inverted wave/Special search/Check Value1 ==
  buf : Inport
  idx : Inport  Port=2
  Abs : Abs
  Compare To Zero : simulink/Logic and Bit Operations/Compare To Zero  relop=<  OutDataTypeStr=boolean
  Constant : Constant  Value=BufferLength
  Selector : Selector  InputPortWidth=BufferLength  IndexOptions=Index vector (port)  Indices=[1 3]
  Sum : Sum  Inputs=|++
  val : Outport
  sign : Outport  Port=2
  wires:
  Selector/1 -> Compare To Zero/1, Abs/1
  Abs/1 -> val/1
  idx/1 -> Sum/1
  buf/1 -> Selector/1
  Constant/1 -> Sum/2
  Compare To Zero/1 -> sign/1
  Sum/1 -> Selector/2

== system model/Preprocessing/Subsystem/FP Detection/Detect R wave points/Search onset and offset/Normal wave/Special search/Check Value ==
  buf : Inport
  idx : Inport  Port=2
  Abs : Abs
  Compare To Zero : simulink/Logic and Bit Operations/Compare To Zero  relop=<  OutDataTypeStr=boolean
  Constant : Constant  Value=BufferLength
  Selector : Selector  InputPortWidth=BufferLength  IndexOptions=Index vector (port)  Indices=[1 3]
  Sum : Sum  Inputs=|++
  val : Outport
  sign : Outport  Port=2
  wires:
  Sum/1 -> Selector/2
  Compare To Zero/1 -> sign/1
  Constant/1 -> Sum/2
  buf/1 -> Selector/1
  idx/1 -> Sum/1
  Abs/1 -> val/1
  Selector/1 -> Abs/1, Compare To Zero/1

== system model/Preprocessing/Subsystem/FP Detection/Detect R wave points/Search onset and offset/Normal wave/Special search/Check Value1 ==
  buf : Inport
  idx : Inport  Port=2
  Abs : Abs
  Compare To Zero : simulink/Logic and Bit Operations/Compare To Zero  relop=<  OutDataTypeStr=boolean
  Constant : Constant  Value=BufferLength
  Selector : Selector  InputPortWidth=BufferLength  IndexOptions=Index vector (port)  Indices=[1 3]
  Sum : Sum  Inputs=|++
  val : Outport
  sign : Outport  Port=2
  wires:
  Selector/1 -> Compare To Zero/1, Abs/1
  Abs/1 -> val/1
  idx/1 -> Sum/1
  buf/1 -> Selector/1
  Constant/1 -> Sum/2
  Compare To Zero/1 -> sign/1
  Sum/1 -> Selector/2
